simulink model "HDLDemodSep"  (R2024a)
settings: Solver=FixedStepDiscrete  StartTime=0.0  StopTime=stopTime  RelTol=1e-3
model workspace (MAT data in the model file):
  RxTree : serdes.internal.ibisami.ami.SerDesTree (value not decoded)
undefined symbols (not defined in the file or in its folder): CONST
libraries: dspsrcs4 x5, HDL_ieee_8021513 x5, whdlutilities x2, hdlsllib x1
settings Model: DataTypeOverride=Off  Creator=cotti  LastModifiedBy=cotti
settings OptimizationCC: BlockReduction=off  ConditionallyExecuteInputs=off  DefaultParameterBehavior=Inlined  InheritOutputTypeSmallerThanSingle=on
settings DebuggingCC: AlgebraicLoopMsg=error  ArtificialAlgebraicLoopMsg=error  SingleTaskRateTransMsg=error  UnconnectedInputMsg=warning  UnconnectedOutputMsg=warning  UnconnectedLineMsg=warning
settings HardwareCC: ProdBitPerPointer=32  ProdBitPerSizeT=32  ProdBitPerPtrDiffT=32  ProdLargestAtomicFloat=None  ProdIntDivRoundTo=Undefined  ProdEndianess=Unspecified  ProdWordSize=32  ProdHWDeviceType=ASIC/FPGA->ASIC/FPGA  TargetBitPerLong=64  TargetBitPerPointer=64  TargetBitPerSizeT=64  TargetBitPerPtrDiffT=64  TargetLongLongMode=on  TargetIntDivRoundTo=Zero  TargetEndianess=LittleEndian  TargetWordSize=64  TargetHWDeviceType=Custom Processor->MATLAB Host Computer  ProdEqTarget=off

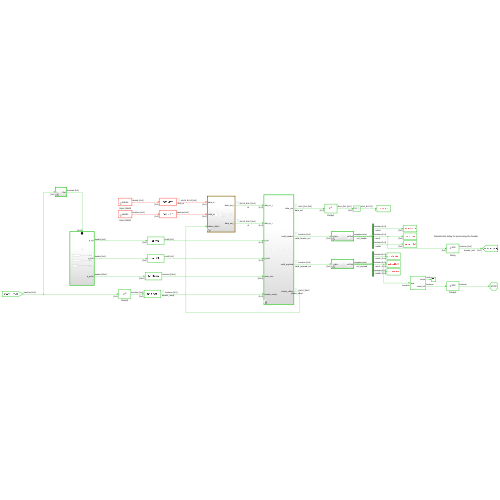
[thumbnail: Simulink's stored preview of the top-level diagram]
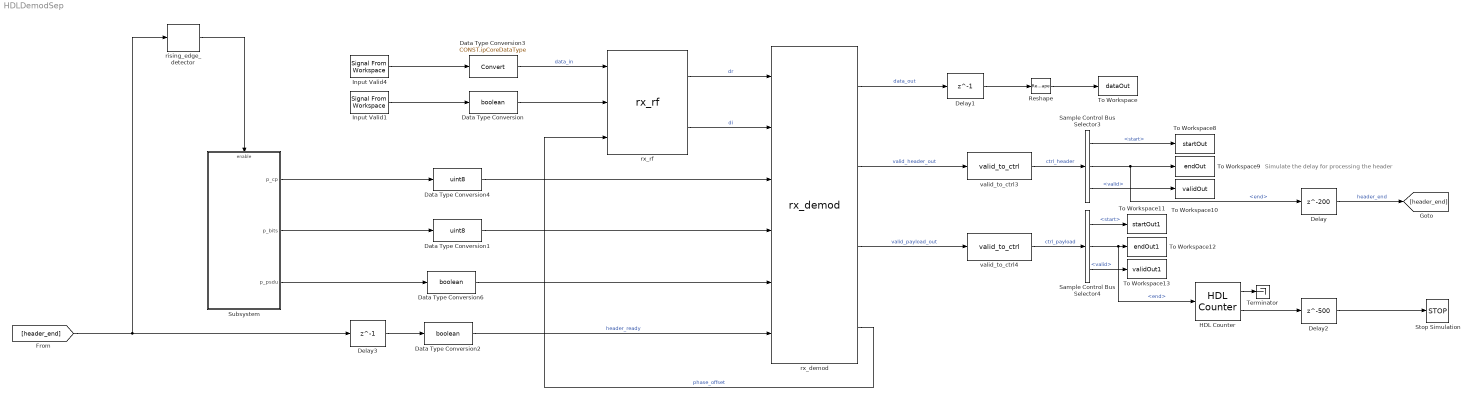
== system HDLDemodSep ==
  note: Simulate the delay for processing the header
  Data Type Conversion : DataTypeConversion  OutDataTypeStr=boolean  SaturateOnIntegerOverflow=off  RndMeth=Floor
  Data Type Conversion1 : DataTypeConversion  OutDataTypeStr=uint8  SaturateOnIntegerOverflow=off  RndMeth=Floor
  Data Type Conversion2 : DataTypeConversion  OutDataTypeStr=boolean  SaturateOnIntegerOverflow=off  RndMeth=Floor
  Data Type Conversion3 : DataTypeConversion  OutDataTypeStr=CONST.ipCoreDataType  SaturateOnIntegerOverflow=off  RndMeth=Floor
  Data Type Conversion4 : DataTypeConversion  OutDataTypeStr=uint8  SaturateOnIntegerOverflow=off  RndMeth=Floor
  Data Type Conversion6 : DataTypeConversion  OutDataTypeStr=boolean  SaturateOnIntegerOverflow=off  RndMeth=Floor
  Delay : Delay  DelayLength=200  InitialCondition=0  UseCircularBuffer=on
  Delay1 : Delay  DelayLength=1  InitialCondition=0  UseCircularBuffer=on
  Delay2 : Delay  DelayLength=500  InitialCondition=0  UseCircularBuffer=on
  Delay3 : Delay  DelayLength=1  InitialCondition=0  UseCircularBuffer=on
  HDL Counter : hdlsllib/Sources/HDL Counter  CountType=Count limited  CountInit=0  CountStep=1  CountMax=totalOFDMSymbols  CountFromType=Initial value  CountFrom=0  CountResetPort=off  CountLoadPort=off  CountEnbPort=on  CountDirPort=off  CountHitOutputPort=on  CountDataType=Unsigned  CountWordLen=8  CountFracLen=0  CountSampTime=1
  Input Valid1 : dspsrcs4/Signal From Workspace  X=validIn  Ts=1/CONST.fADC  nsamps=1  OutputAfterFinalValue=Setting to zero  ignoreOrWarnInputAndFrameLengths=off  OutputFrames=off
  Input Valid4 : dspsrcs4/Signal From Workspace  X=dataIn  Ts=1/CONST.fADC  nsamps=1  OutputAfterFinalValue=Setting to zero  ignoreOrWarnInputAndFrameLengths=off  OutputFrames=off
  Reshape : Reshape
  Sample Control Bus Selector3 : whdlutilities/Sample Control Bus Selector  OutputSignals=start,end,valid
  Sample Control Bus Selector4 : whdlutilities/Sample Control Bus Selector  OutputSignals=start,end,valid
  Stop Simulation : Stop
  Subsystem : Subsystem
  Terminator : Terminator
  To Workspace : ToWorkspace  VariableName=dataOut  SampleTime=1/CONST.fPHY
      settings: Save2DSignal=2-D array (concatenate along first dimension)
  To Workspace10 : ToWorkspace  VariableName=validOut  SampleTime=1/CONST.fPHY
      settings: Save2DSignal=2-D array (concatenate along first dimension)
  To Workspace11 : ToWorkspace  VariableName=startOut1  SampleTime=1/CONST.fPHY
      settings: Save2DSignal=2-D array (concatenate along first dimension)
  To Workspace12 : ToWorkspace  VariableName=endOut1  SampleTime=1/CONST.fPHY
      settings: Save2DSignal=2-D array (concatenate along first dimension)
  To Workspace13 : ToWorkspace  VariableName=validOut1  SampleTime=1/CONST.fPHY
      settings: Save2DSignal=2-D array (concatenate along first dimension)
  To Workspace8 : ToWorkspace  VariableName=startOut  SampleTime=1/CONST.fPHY
      settings: Save2DSignal=2-D array (concatenate along first dimension)
  To Workspace9 : ToWorkspace  VariableName=endOut  SampleTime=1/CONST.fPHY
      settings: Save2DSignal=2-D array (concatenate along first dimension)
  rising_edge_detector : HDL_ieee_8021513/rising_edge_detector  SystemSampleTime=-1  VariantActivationTime=update diagram  AllowFlexibleInterface=on  Latency=0  AutoFrameSizeCalculation=off
      settings: SourceProductName=HDL IEEE 8021513
  rx_demod : HDL_ieee_8021513/rx_demod  SystemSampleTime=-1  VariantActivationTime=update diagram  AllowFlexibleInterface=on  Latency=0  AutoFrameSizeCalculation=off
      settings: SourceProductName=HDL IEEE 8021513
  rx_rf : HDL_ieee_8021513/rx_rf  SystemSampleTime=-1  VariantActivationTime=update diagram  AllowFlexibleInterface=on  Latency=0  AutoFrameSizeCalculation=off
      settings: SourceProductName=HDL IEEE 8021513
  valid_to_ctrl3 : HDL_ieee_8021513/valid_to_ctrl  SystemSampleTime=-1  VariantActivationTime=update diagram  AllowFlexibleInterface=on  Latency=0  AutoFrameSizeCalculation=off
      settings: SourceProductName=HDL IEEE 8021513
  valid_to_ctrl4 : HDL_ieee_8021513/valid_to_ctrl  SystemSampleTime=-1  VariantActivationTime=update diagram  AllowFlexibleInterface=on  Latency=0  AutoFrameSizeCalculation=off
      settings: SourceProductName=HDL IEEE 8021513
  wires:
  rx_rf/1 -> rx_demod/1  "dr"
  rx_rf/2 -> rx_demod/2  "di"
  rx_demod/4 -> rx_rf/3  "phase_offset"
  HDL Counter/2 -> Delay2/1
  valid_to_ctrl3/1 -> Sample Control Bus Selector3/1  "ctrl_header"
  Delay2/1 -> Stop Simulation/1
  Sample Control Bus Selector3/2 -> Delay/1, To Workspace9/1  "<end>"
  Sample Control Bus Selector3/1 -> To Workspace8/1  "<start>"
  Reshape/1 -> To Workspace/1
  rx_demod/1 -> Delay1/1  "data_out"
  Delay/1 -> [header_end]  "header_end"
  valid_to_ctrl4/1 -> Sample Control Bus Selector4/1  "ctrl_payload"
  Sample Control Bus Selector4/2 -> HDL Counter/1, To Workspace12/1  "<end>"
  Sample Control Bus Selector3/3 -> To Workspace10/1  "<valid>"
  rx_demod/3 -> valid_to_ctrl4/1  "valid_payload_out"
  Delay1/1 -> Reshape/1
  rx_demod/2 -> valid_to_ctrl3/1  "valid_header_out"
  HDL Counter/1 -> Terminator/1
  Sample Control Bus Selector4/1 -> To Workspace11/1  "<start>"
  Sample Control Bus Selector4/3 -> To Workspace13/1  "<valid>"
  Delay3/1 -> Data Type Conversion2/1
  Subsystem/3(p_psdu) -> Data Type Conversion6/1
  [header_end] -> rising_edge_detector/1, Delay3/1
  Subsystem/1(p_cp) -> Data Type Conversion4/1
  Data Type Conversion2/1 -> rx_demod/6  "header_ready"
  Data Type Conversion3/1 -> rx_rf/1  "data_in"
  Subsystem/2(p_bits) -> Data Type Conversion1/1
  Input Valid4/1 -> Data Type Conversion3/1
  rising_edge_detector/1 -> Subsystem/Enable
  Data Type Conversion4/1 -> rx_demod/3
  Data Type Conversion1/1 -> rx_demod/4
  Data Type Conversion6/1 -> rx_demod/5
  Input Valid1/1 -> Data Type Conversion/1
  Data Type Conversion/1 -> rx_rf/2

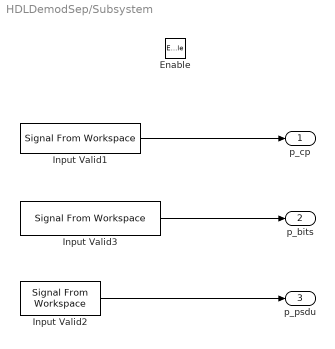
== system HDLDemodSep/Subsystem ==
  Enable : EnablePort
  Input Valid1 : dspsrcs4/Signal From Workspace  X=payloadCyclicPrefixLenIn  Ts=1/CONST.fPHY  nsamps=1  OutputAfterFinalValue=Setting to zero  ignoreOrWarnInputAndFrameLengths=off  OutputFrames=off
  Input Valid2 : dspsrcs4/Signal From Workspace  X=psduSizeLSB  Ts=1/CONST.fPHY  nsamps=1  OutputAfterFinalValue=Setting to zero  ignoreOrWarnInputAndFrameLengths=off  OutputFrames=off
  Input Valid3 : dspsrcs4/Signal From Workspace  X=payloadBitsPerSubcarrierIn  Ts=1/CONST.fPHY  nsamps=1  OutputAfterFinalValue=Setting to zero  ignoreOrWarnInputAndFrameLengths=off  OutputFrames=off
  p_cp : Outport
  p_bits : Outport  Port=2
  p_psdu : Outport  Port=3
  wires:
  Input Valid2/1 -> p_psdu/1
  Input Valid1/1 -> p_cp/1
  Input Valid3/1 -> p_bits/1
